simulink model "Stabilizer_QBot2_r2018a"  (Simulink 9.1)
settings: Solver=ode2  StartTime=0.0  StopTime=inf  FixedStep=0.001  RelTol=1e-3  EnableMultiTasking=on
model workspace (MAT data in the model file):
  Sig = Simulink.Signal
  Sig.DataType = 'auto'
  Sig.Dimensions = -1
  Sig.DimensionsMode = 'auto'
  Sig.Complexity = 'auto'
  Sig.SampleTime = -1
  Sig.SamplingMode = 'auto'
  video_step_size = 0.06
undefined symbols (not defined in the file): HIL
libraries: quarc_library x14
settings Model: Creator=Admin  LastModifiedBy=user  SimulationMode=external
settings SolverCC: PositivePriorityOrder=on
settings DataIOCC: SaveFormat=Dataset
settings OptimizationCC: LifeSpan=auto
settings DebuggingCC: UnderspecifiedInitializationDetection=Simplified  MergeDetectMultiDrivingBlocksExec=error  ParameterPrecisionLossMsg=none
settings HardwareCC: ProdLargestAtomicInteger=Long  ProdLargestAtomicFloat=Double  ProdIntDivRoundTo=Zero  ProdEndianess=LittleEndian  ProdHWDeviceType=ARM Compatible->ARM Cortex
settings ModelReferenceCC: PropagateSignalLabelsOutOfModel=on
settings RTWCC: Description=QUARC Linux DuoVero 2016 Target (QBall 2, QBot 2) Using Toolchain  SystemTargetFile=quarc_linux_duovero_2016.tlc  TemplateMakefile=quarc_default_tmf  Toolchain=QUARC linux_duovero_2016 | gmake (64-bit Windows)  BuildConfiguration=Faster Runs
settings STFCustomTargetCC: ConcurrentExecutionCompliant=on  UseToolchainInfoCompliant=on  SystemTargetFile=quarc_linux_duovero_2016.tlc
settings GRTTargetCC: ParMdlRefBuildCompliant=off  CompOptLevelCompliant=off  MatFileLogging=off  CPPClassGenCompliant=off  ExtMode=on  ExtModeMexFile=quarc_comm  ExtModeMexArgs='-w -d /tmp -uri %u -URI_Host tcpip://192.168.2.H:18000','tcpip://192.168.2.X:17001'

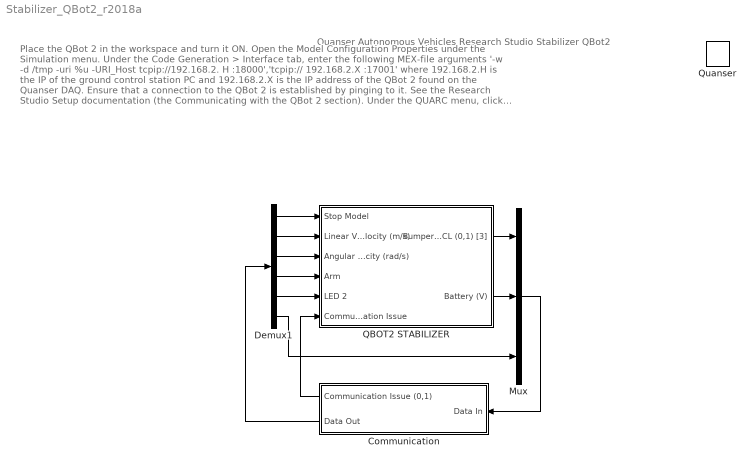
== system Stabilizer_QBot2_r2018a ==
  note: Quanser Autonomous Vehicles Research Studio
      | Stabilizer QBot2
  note: Place the QBot 2 in the workspace and turn it ON.
      |
      | Open the Model Configuration Properties under the Simulation menu.
      |
      | Under the Code Generation > Interface tab, enter the following MEX-file arguments
      | '-w -d /tmp -uri %u -URI_Host tcpip://192.168.2. H :18000','tcpip:// 192.168.2.X :17001'
      | where 192.168.2.H is the IP of the ground control station PC and 192.168.2.X is the IP address of the QBot 2 found on the Quanser DAQ.
      |
      | Ensure that a connection to the QBot 2 is established by pinging to it. See the Research Studio Setup documentation (the Communicating with the QBot 2 section).
      |
      | Under the QUARC menu, click on Build .
      | NOTE : Ensure that the corresponding Mission_Server_QBot2_IO_Check is running first before continuing.
      |
      | Under the QUARC menu, click on Start .
      |
      | You will hear a sequence of beeps, which indicate that the model has started running on the QBot.
      |
      | Confirm proper operation of the QBot 2 and once complete, stop this model.
      | NOTE : This model will terminate automatically if not communicating with the Mission_Server_QBot2_IO_Check model runnning on the ground control station PC.
  Communication : Subsystem
  Demux1 : Demux  Outputs=6
  Mux : Mux  Inputs=3
  QBOT2 STABILIZER : Subsystem
  Quanser : quarc_library/Logos/Quanser
  wires:
  Demux1/6 -> Mux/3
  Mux/1 -> Communication/1(Data In)
  Communication/2(Data Out) -> Demux1/1
  QBOT2 STABILIZER/1(Bumpers - RCL (0,1) [3]) -> Mux/1
  QBOT2 STABILIZER/2(Battery (V)) -> Mux/2
  Demux1/1 -> QBOT2 STABILIZER/1(Stop Model)
  Demux1/2 -> QBOT2 STABILIZER/2(Linear Velocity (m/s))
  Demux1/3 -> QBOT2 STABILIZER/3(Angular Velocity (rad/s))
  Demux1/4 -> QBOT2 STABILIZER/4(Arm)
  Demux1/5 -> QBOT2 STABILIZER/5(LED 2)
  Communication/1(Communication Issue (0,1)) -> QBOT2 STABILIZER/6(Communication Issue)

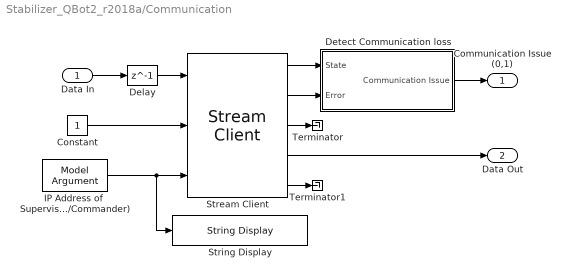
== system Stabilizer_QBot2_r2018a/Communication ==
  Data In : Inport
  Constant : Constant
  Delay : Delay  DelayLength=1
  Detect Communication loss : Subsystem
  IP Address of  Supervisory Model (Mission Operator/Commander) : quarc_library/Sources/Signals/Model Argument  argument_name=URI_Host  has_value=on  data_type_mode=Specify via dialog  data_type=char  max_length=80  default_value=0  variable_size=off
      settings: AttributesFormatString=(-%<argument_name>)  SourceProductName=QUARC Targets
  Stream Client : quarc_library/Communications/Basic/Stream Client  uri_source=External input port  uri=tcpip://localhost:18999  apply_uri_to_all_configs=on  send_buffer_size=1460  receive_buffer_size=1460  byte_order=little endian (Intel - LSB first)  optimization=Minimum latency  send_options=Send most recent data  receive_options=Receive most recent data  default_value=zeros(1,6)  sample_time=qc_get_step_size  active=off  implementation=Use blocking I/O in a separate thread  send_fifo_size=1  receive_fifo_size=1  send_priority=0  receive_priority=0  send_dimensions=off  receive_dimensions=off  max_dimensions=-1  data_type=Inherited via back propagation  type_expr=BusObject
      settings: SourceProductName=The database C:\Users\user\AppData\Roaming\MathWorks\MATLAB\R2017a\slblocks_master.db is locked, or a table in the database is locked. (database is locked)
  String Display : quarc_library/Strings/String Display  alignment=center  display_mode=Single line  sample_time=-1  use_new=off
      settings: SourceProductName=QUARC Targets
  Terminator : Terminator
  Terminator1 : Terminator
  Communication Issue (0,1) : Outport  VectorParamsAs1DForOutWhenUnconnected=off
  Data Out : Outport  Port=2  VectorParamsAs1DForOutWhenUnconnected=off
  wires:
  Stream Client/5 -> Terminator1/1
  Constant/1 -> Stream Client/2
  Stream Client/3 -> Terminator/1
  IP Address of  Supervisory Model (Mission Operator/Commander)/1 -> Stream Client/3, String Display/1
  Stream Client/1 -> Detect Communication loss/1(State)
  Stream Client/2 -> Detect Communication loss/2(Error)
  Stream Client/4 -> Data Out/1
  Data In/1 -> Delay/1
  Delay/1 -> Stream Client/1
  Detect Communication loss/1(Communication Issue) -> Communication Issue (0,1)/1

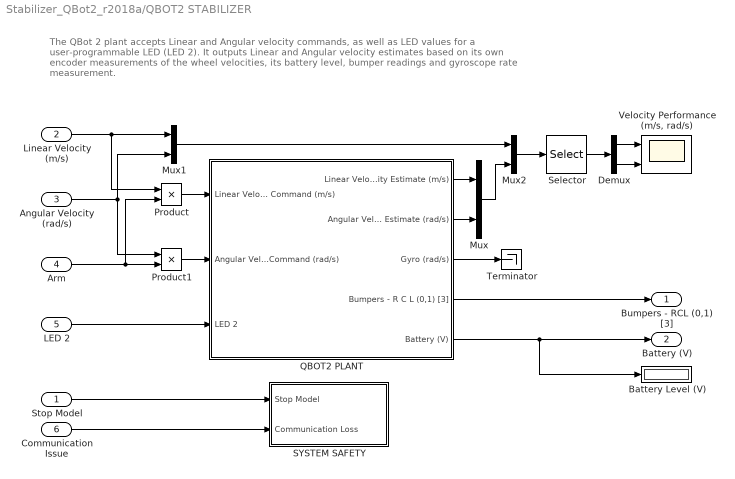
== system Stabilizer_QBot2_r2018a/QBOT2 STABILIZER ==
  note: The QBot 2 plant accepts Linear and Angular velocity commands, as well as LED values for a user-programmable LED (LED 2).
      | It outputs Linear and Angular velocity estimates based on its own encoder measurements of the wheel velocities, its battery level,
      | bumper readings and gyroscope rate measurement.
  Stop Model : Inport
  Linear Velocity (m/s) : Inport  Port=2
  Angular Velocity (rad/s) : Inport  Port=3
  Arm : Inport  Port=4
  LED 2 : Inport  Port=5
  Communication Issue : Inport  Port=6
  Battery Level (V) : Display
  Demux : Demux  Outputs=[2 2]
  Mux : Mux  Inputs=2
  Mux1 : Mux  Inputs=2
  Mux2 : Mux  Inputs=2
  Product : Product
  Product1 : Product
  QBOT2 PLANT : Subsystem
  SYSTEM SAFETY : Subsystem
  Selector : Selector  InputPortWidth=4  IndexOptions=Index vector (dialog)  Indices=[1 3 2 4]  OutputSizes=1
  Terminator : Terminator
  "Velocity Performance (m/s, rad/s)" : Scope  NumInputPorts=2
  Bumpers - RCL (0,1) [3] : Outport  VectorParamsAs1DForOutWhenUnconnected=off
  Battery (V) : Outport  Port=2  VectorParamsAs1DForOutWhenUnconnected=off
  wires:
  Angular Velocity (rad/s)/1 -> Product1/1, Mux1/2
  Linear Velocity (m/s)/1 -> Product/1, Mux1/1
  Mux1/1 -> Mux2/1
  Mux2/1 -> Selector/1
  Selector/1 -> Demux/1
  Demux/1 -> "Velocity Performance (m/s, rad/s)"/1
  Demux/2 -> "Velocity Performance (m/s, rad/s)"/2
  Arm/1 -> Product1/2, Product/2
  Stop Model/1 -> SYSTEM SAFETY/1(Stop Model)
  Communication Issue/1 -> SYSTEM SAFETY/2(Communication Loss)
  Product1/1 -> QBOT2 PLANT/2(Angular Velocity Command (rad/s))
  Product/1 -> QBOT2 PLANT/1(Linear Velocity Command (m/s))
  LED 2/1 -> QBOT2 PLANT/3(LED 2)
  QBOT2 PLANT/5(Battery (V)) -> Battery Level (V)/1, Battery (V)/1
  QBOT2 PLANT/4(Bumpers - R C L (0,1) [3]) -> Bumpers - RCL (0,1) [3]/1
  QBOT2 PLANT/2(Angular Velocity Estimate (rad/s)) -> Mux/2
  QBOT2 PLANT/1(Linear Velocity Estimate (m/s)) -> Mux/1
  Mux/1 -> Mux2/2
  QBOT2 PLANT/3(Gyro (rad/s)) -> Terminator/1

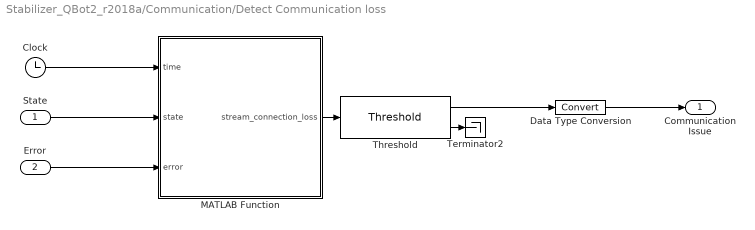
== system Stabilizer_QBot2_r2018a/Communication/Detect Communication loss ==
  State : Inport
  Error : Inport  Port=2
  Clock : Clock
  Data Type Conversion : DataTypeConversion
  MATLAB Function : MATLAB Function  TreatAsAtomicUnit=on
  Terminator2 : Terminator
  Threshold : quarc_library/Discontinuities/Threshold  operator=>=  param_src=Specify via dialog  threshold=0.5  duration=0.1
      settings: SourceProductName=QUARC Targets
  Communication Issue : Outport  VectorParamsAs1DForOutWhenUnconnected=off
  wires:
  Error/1 -> MATLAB Function/3(error)
  MATLAB Function/1(stream_connection_loss) -> Threshold/1
  State/1 -> MATLAB Function/2(state)
  Clock/1 -> MATLAB Function/1(time)
  Threshold/1 -> Data Type Conversion/1
  Threshold/2 -> Terminator2/1
  Data Type Conversion/1 -> Communication Issue/1

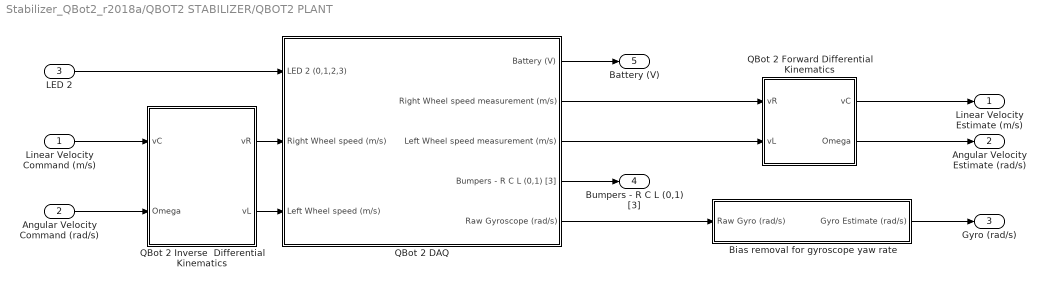
== system Stabilizer_QBot2_r2018a/QBOT2 STABILIZER/QBOT2 PLANT ==
  Linear Velocity Command (m/s) : Inport
  Angular Velocity Command (rad/s) : Inport  Port=2
  LED 2 : Inport  Port=3
  Bias removal for gyroscope yaw rate : Subsystem
  QBot 2 DAQ : Subsystem
  QBot 2 Forward Differential Kinematics : MATLAB Function  TreatAsAtomicUnit=on
  QBot 2 Inverse  Differential Kinematics : MATLAB Function  TreatAsAtomicUnit=on
  Linear Velocity Estimate (m/s) : Outport  VectorParamsAs1DForOutWhenUnconnected=off
  Angular Velocity Estimate (rad/s) : Outport  Port=2  VectorParamsAs1DForOutWhenUnconnected=off
  Gyro (rad/s) : Outport  Port=3  VectorParamsAs1DForOutWhenUnconnected=off
  Bumpers - R C L (0,1) [3] : Outport  Port=4  VectorParamsAs1DForOutWhenUnconnected=off
  Battery (V) : Outport  Port=5  VectorParamsAs1DForOutWhenUnconnected=off
  wires:
  Angular Velocity Command (rad/s)/1 -> QBot 2 Inverse  Differential Kinematics/2(Omega)
  Linear Velocity Command (m/s)/1 -> QBot 2 Inverse  Differential Kinematics/1(vC)
  QBot 2 Forward Differential Kinematics/1(vC) -> Linear Velocity Estimate (m/s)/1
  QBot 2 Forward Differential Kinematics/2(Omega) -> Angular Velocity Estimate (rad/s)/1
  Bias removal for gyroscope yaw rate/1(Gyro Estimate (rad/s)) -> Gyro (rad/s)/1
  LED 2/1 -> QBot 2 DAQ/1(LED 2 (0,1,2,3))
  QBot 2 Inverse  Differential Kinematics/1(vR) -> QBot 2 DAQ/2(Right Wheel speed (m/s))
  QBot 2 Inverse  Differential Kinematics/2(vL) -> QBot 2 DAQ/3(Left Wheel speed (m/s))
  QBot 2 DAQ/1(Battery (V)) -> Battery (V)/1
  QBot 2 DAQ/2(Right Wheel speed measurement (m/s)) -> QBot 2 Forward Differential Kinematics/1(vR)
  QBot 2 DAQ/3(Left Wheel speed measurement (m/s)) -> QBot 2 Forward Differential Kinematics/2(vL)
  QBot 2 DAQ/4(Bumpers - R C L (0,1) [3]) -> Bumpers - R C L (0,1) [3]/1
  QBot 2 DAQ/5(Raw Gyroscope (rad/s)) -> Bias removal for gyroscope yaw rate/1(Raw Gyro (rad/s))

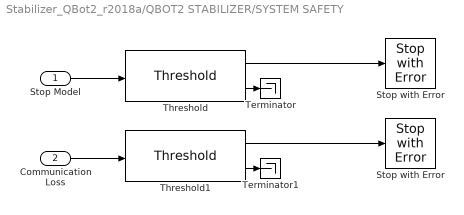
== system Stabilizer_QBot2_r2018a/QBOT2 STABILIZER/SYSTEM SAFETY ==
  Stop Model : Inport
  Communication Loss : Inport  Port=2
  Stop with Error : quarc_library/Sinks/Error Handling/Stop with Error  message_type=Fixed error message  message=QBot 2 Stabilizer: Operator Stopped Model
      settings: AttributesFormatString="\"%<message>\""  SourceProductName=QUARC Targets
  "Stop with Error " : quarc_library/Sinks/Error Handling/Stop with Error  message_type=Fixed error message  message=QBot 2 Stabilizer: Communication Issue with Operator
      settings: AttributesFormatString="\"%<message>\""  SourceProductName=QUARC Targets
  Terminator : Terminator
  Terminator1 : Terminator
  Threshold : quarc_library/Discontinuities/Threshold  operator=>  param_src=Specify via dialog  threshold=0.5  duration=2
      settings: SourceProductName=QUARC Targets
  Threshold1 : quarc_library/Discontinuities/Threshold  operator=>  param_src=Specify via dialog  threshold=0.5  duration=3
      settings: SourceProductName=QUARC Targets
  wires:
  Threshold/1 -> Stop with Error/1
  Communication Loss/1 -> Threshold1/1
  Threshold1/1 -> "Stop with Error "/1
  Threshold1/2 -> Terminator1/1
  Stop Model/1 -> Threshold/1
  Threshold/2 -> Terminator/1

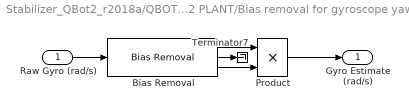
== system Stabilizer_QBot2_r2018a/QBOT2 STABILIZER/QBOT2 PLANT/Bias removal for gyroscope yaw rate ==
  Raw Gyro (rad/s) : Inport
  Bias Removal : quarc_library/Discrete/Bias Removal  start_time=3  end_time=4  switch_id=0  sample_time=qc_get_step_size
      settings: SourceProductName=QUARC Targets
  Product : Product  RndMeth=Zero
  Terminator7 : Terminator
  Gyro Estimate (rad/s) : Outport  VectorParamsAs1DForOutWhenUnconnected=off
  wires:
  Bias Removal/3 -> Product/2
  Bias Removal/2 -> Terminator7/1
  Raw Gyro (rad/s)/1 -> Bias Removal/1
  Product/1 -> Gyro Estimate (rad/s)/1
  Bias Removal/1 -> Product/1

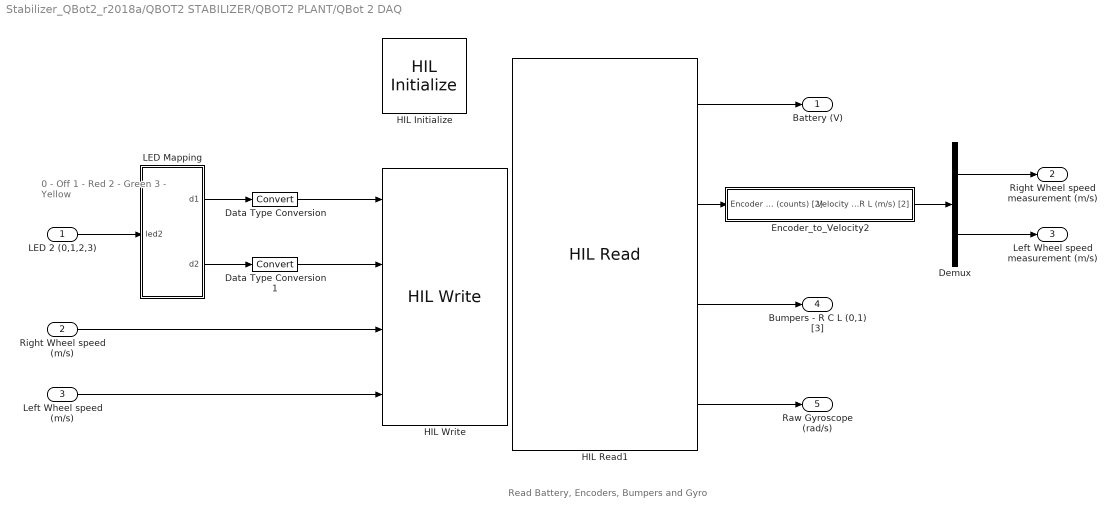
== system Stabilizer_QBot2_r2018a/QBOT2 STABILIZER/QBOT2 PLANT/QBot 2 DAQ ==
  note: 0 - Off
      | 1 - Red
      | 2 - Green
      | 3 - Yellow
  note: Read Battery, Encoders, Bumpers and Gyro
  LED 2 (0,1,2,3) : Inport
  Right Wheel speed (m/s) : Inport  Port=2
  Left Wheel speed (m/s) : Inport  Port=3
  Data Type Conversion : DataTypeConversion
  Data Type Conversion1 : DataTypeConversion
  Demux : Demux  Outputs=2
  Encoder_to_Velocity2 : Subsystem
  HIL Initialize : quarc_library/Data Acquisition/Generic/Configuration/HIL Initialize  Priority=-99  object_name=HIL-1  board_type=qbot2  board_number=0  board_options=enc0_dir=0;enc0_filter=1;enc0_a=0;enc0_b=0;enc0_z=1;enc0_reload=0;enc1_dir=0;enc1_filter=1;enc1_a=0;enc1_b=0;enc1_z=1;enc1_reload=0;pwm0_immediate=0;pwm1_immediate=0;pwm2_immediate=0;pwm3_immediate=0;  exclusive=off  active=off  hardware_clocks=[]  clock_modes=[]  initial_clock_frequencies=[]  set_clock_params_at_start=off  set_clock_params_at_switch_in=off  set_clock_frequencies_at_start=off  set_clock_frequencies_at_switch_in=off  analog_input_channels=[0:9]  analog_input_configurations=0  analog_input_maximums=[5 5 5 5 16.5 3.3 3.3 3.3 3.3]  analog_input_minimums=[0 0 0 0 0 0 0 0 0]  set_analog_input_params_at_start=off  set_analog_input_params_at_switch_in=off  analog_output_channels=[]  analog_output_maximums=[]  analog_output_minimums=[]  initial_analog_outputs=[]  final_analog_outputs=[]  watchdog_analog_outputs=[]  set_analog_output_params_at_start=off  set_analog_output_params_at_switch_in=off  set_analog_outputs_at_start=off  set_analog_outputs_at_switch_in=off  set_analog_outputs_at_terminate=off  set_analog_outputs_at_switch_out=off  set_analog_outputs_on_watchdog=off  digital_input_channels=[]  digital_output_channels=[9:12]  digital_output_configuration=[]  initial_digital_outputs=[0]  final_digital_outputs=[0]  watchdog_digital_outputs=[0]  set_digital_output_params_at_start=off  set_digital_output_params_at_switch_in=off  set_digital_outputs_at_start=on  set_digital_outputs_at_switch_in=off  set_digital_outputs_at_terminate=on  set_digital_outputs_at_switch_out=off  set_digital_outputs_on_watchdog=on  encoder_channels=[0:3]  quadrature=[4]  encoder_filter_frequency=[]  initial_encoder_counts=[0]  set_encoder_params_at_start=on  set_encoder_params_at_switch_in=off  set_encoder_counts_at_start=on  set_encoder_counts_at_switch_in=off  pwm_channels=[0:3]  pwm_modes=[0]  pwm_frequency=[20e6/1024]  pwm_configuration=[0]  pwm_alignment=[0]  pwm_polarity=[1]  pwm_leading_deadband=[0]  pwm_trailing_deadband=[0]  initial_pwm_outputs=[0]  final_pwm_outputs=[0]  watchdog_pwm_outputs=[0]  set_pwm_params_at_start=on  set_pwm_params_at_switch_in=off  set_pwm_outputs_at_start=on  set_pwm_outputs_at_switch_in=off  set_pwm_outputs_at_terminate=on  set_pwm_outputs_at_switch_out=off  set_pwm_outputs_on_watchdog=on  other_output_channels=[2000:2001 14000 16000]  initial_other_outputs=[0 0 0 7]  final_other_outputs=[0 0 0 7]  watchdog_other_outputs=[]  set_other_outputs_at_start=on  set_other_outputs_at_switch_in=off  set_other_outputs_at_terminate=on  set_other_outputs_at_switch_out=off  set_other_outputs_on_watchdog=off
  HIL Read1 : quarc_library/Data Acquisition/Generic/Immediate I//O/HIL Read  object_name=HIL-1  analog_channels=[4]  encoder_channels=[2 3]  digital_channels=[8 9 10]  other_channels=[1002]  sample_time=qc_get_step_size  active=on  vector_output=on  data_type_mode=Inherit via back propagation  encoder_data_type=double  digital_data_type=boolean
  HIL Write : quarc_library/Data Acquisition/Generic/Immediate I//O/HIL Write  object_name=HIL-1  analog_channels=[]  pwm_channels=[]  digital_channels=[11:12]  other_channels=[2000:2001]  sample_time=-1  active=on  vector_input=off
  LED Mapping : MATLAB Function  TreatAsAtomicUnit=on
  Battery (V) : Outport  VectorParamsAs1DForOutWhenUnconnected=off
  Right Wheel speed measurement (m/s) : Outport  Port=2  VectorParamsAs1DForOutWhenUnconnected=off
  Left Wheel speed measurement (m/s) : Outport  Port=3  VectorParamsAs1DForOutWhenUnconnected=off
  Bumpers - R C L (0,1) [3] : Outport  Port=4  VectorParamsAs1DForOutWhenUnconnected=off
  Raw Gyroscope (rad/s) : Outport  Port=5  VectorParamsAs1DForOutWhenUnconnected=off
  wires:
  HIL Read1/3 -> Bumpers - R C L (0,1) [3]/1
  LED Mapping/1(d1) -> Data Type Conversion/1
  Right Wheel speed (m/s)/1 -> HIL Write/3
  Data Type Conversion1/1 -> HIL Write/2
  HIL Read1/2 -> Encoder_to_Velocity2/1(Encoder - R L (counts) [2])
  LED Mapping/2(d2) -> Data Type Conversion1/1
  Encoder_to_Velocity2/1(Velocity - R L (m/s) [2]) -> Demux/1
  LED 2 (0,1,2,3)/1 -> LED Mapping/1(led2)
  Data Type Conversion/1 -> HIL Write/1
  Demux/1 -> Right Wheel speed measurement (m/s)/1
  Demux/2 -> Left Wheel speed measurement (m/s)/1
  Left Wheel speed (m/s)/1 -> HIL Write/4
  HIL Read1/1 -> Battery (V)/1
  HIL Read1/4 -> Raw Gyroscope (rad/s)/1

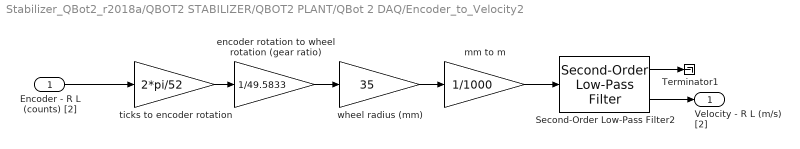
== system Stabilizer_QBot2_r2018a/QBOT2 STABILIZER/QBOT2 PLANT/QBot 2 DAQ/Encoder_to_Velocity2 ==
  Encoder - R L (counts) [2] : Inport
  " encoder rotation to wheel rotation (gear ratio)" : Gain  Gain=1/49.5833
  Second-Order Low-Pass Filter2 : quarc_library/Continuous/Second-Order Low-Pass Filter  params_source=Internal (dialog parameters)  input_width=10  input_zeta=1  input_init=0
  Terminator1 : Terminator
  mm to m : Gain  Gain=1/1000
  ticks to encoder rotation : Gain  Gain=2*pi/52
  wheel radius (mm) : Gain  Gain=35
  Velocity - R L (m/s) [2] : Outport  VectorParamsAs1DForOutWhenUnconnected=off
  wires:
  Second-Order Low-Pass Filter2/1 -> Terminator1/1
  mm to m/1 -> Second-Order Low-Pass Filter2/1
  Second-Order Low-Pass Filter2/2 -> Velocity - R L (m/s) [2]/1
  wheel radius (mm)/1 -> mm to m/1
  ticks to encoder rotation/1 -> " encoder rotation to wheel rotation (gear ratio)"/1
  Encoder - R L (counts) [2]/1 -> ticks to encoder rotation/1
  " encoder rotation to wheel rotation (gear ratio)"/1 -> wheel radius (mm)/1

== matlab function QBOT2 STABILIZER/QBOT2 PLANT/QBot 2 DAQ/LED Mapping ==
  data: d1 output double; led2 input double; d2 output double
function [d1, d2] = fcn(led2)

% Default LEDs are both OFF.
d1 = 0;
d2 = 0;

if led2 == 1
    d1 = 1;
elseif led2 == 2
    d2 = 1;
elseif led2 == 3
    d1 = 1;
    d2 = 1;
elseif (led2 > 3)||(led2 < 1)
	d1 = 1;
    d2 = 1;
end

== matlab function QBOT2 STABILIZER/QBOT2 PLANT/QBot 2 Forward Differential Kinematics ==
  data: vR input double; vL input double; vC output double; Omega output double
function [vC,Omega] = qbot_i_d_k(vR,vL)

d= 0.235; % wheel base

vC = 0.5*(vL+vR); 
Omega = (1/d)*(vR-vL);

== matlab function Communication/Detect Communication loss/MATLAB Function ==
  data: time input double; stream_connection_loss output double; state input double; error input double
function stream_connection_loss  = fcn(time, state, error)

stream_connection_loss = 0;
if time > 3
    if ((state ~= 2)&&(error < 0))
        % stream connection is not established correctly
        stream_connection_loss = 1;
    end
end

== matlab function QBOT2 STABILIZER/QBOT2 PLANT/QBot 2 Inverse Differential Kinematics ==
  data: vR output double; vL output double; vC input double; Omega input double
function [vR,vL] = qbot_f_d_k(vC , Omega)

d=0.235; % wheel base

vR = vC + Omega*d/2; % right wheel velocity
vL= vC - Omega*d/2; % left wheel velocity
